simulink model "pv_curves"  (R2024b)
settings: Solver=VariableStepAuto  StartTime=0.0  StopTime=1.0  RelTol=1e-5
libraries: simulink x1, spspowerguiLib x1
settings Model: Creator=jmy  LastModifiedBy=Eng.Abd-Elrhman Saad

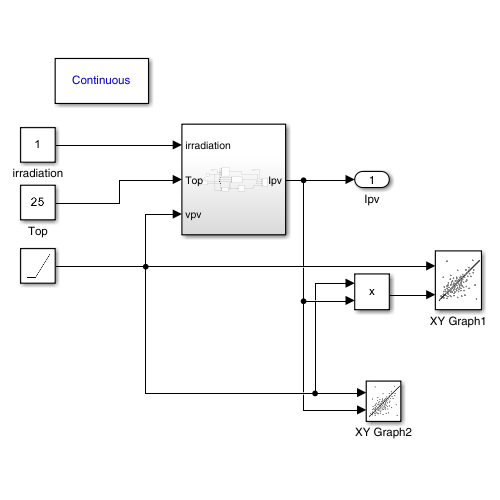
[thumbnail: Simulink's stored preview of the top-level diagram]
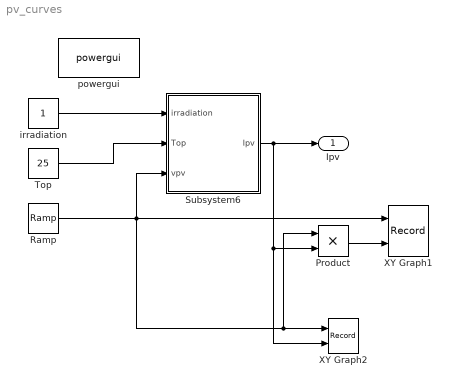
== system pv_curves ==
  Product : Product
  Ramp : simulink/Sources/Ramp  slope=22.9  start=0  InitialOutput=0
  Subsystem6 : Subsystem
  Top : Constant  Value=25
  XY Graph1 : Record  FileSettingsInternal="{\"entries\":[{\"content\":{\"excelSettings\":{\"content\":{},\"type\":\"Streamout.ExcelSettings\"}},\"type\":\"Streamout.FileSettingStorage\",\"uuid\":\"\"}],\"packageUris\":[\"http:\\/\\/schema.mathworks.com\\/mf0\\/streamout_blocks\\/R2020a\"],\"version\":\"1.0\"}"  Layout=[1 1]  SignalsInternal="{\"entries\":[{\"content\":{\"signals\":[{\"content\":{\"blockPath\":[],\"dimensions\":[1],\"domain\":\"\",\"lineColor\":\"#a2142f\",\"plots\":[ 1 ],\"port\":1,\"sid\":[\"\"],\"signalID\":1,\"signalName\":\"Ramp\"},\"type\":\"RecordBlkView.Signal\",\"uuid\":\"\"},{\"content\":{\"blockPath\":[],\"dimensions\":[1],\"domain\":\"\",\"lineColor\":\"#139fff\",\"plots\":[ 1 ],\"port\":2,\"sid\":[\"\"],\"signalID\":2,\"signalName\":\"Product\"},\"type\":\"RecordBlkView.Signal\",\"uuid\":\"\"}]},\"type\":\"RecordBlkView.InputSignals\",\"uuid\":\"\"}],\"packageUris\":[\"http:\\/\\/schema.mathworks.com\\/mf0\\/streamout_blocks\\/R2020a\"],\"version\":\"1.0\"}"  VisualizationBindings="{\"xyplotplugin\":{\"info\":[{\"series\":[{\"bindingParametersList\":[{\"parameter\":\"X-Axis\",\"signalID\":1,\"signalName\":\"Ramp\"},{\"parameter\":\"Y-Axis\",\"signalID\":2,\"signalName\":\"Product\"}],\"seriesID\":0}],\"subplotID\":1}]}}"  CompatibilityTag=XY  st=-1
  XY Graph2 : Record  FileSettingsInternal="{\"entries\":[{\"content\":{\"excelSettings\":{\"content\":{},\"type\":\"Streamout.ExcelSettings\"}},\"type\":\"Streamout.FileSettingStorage\",\"uuid\":\"\"}],\"packageUris\":[\"http:\\/\\/schema.mathworks.com\\/mf0\\/streamout_blocks\\/R2020a\"],\"version\":\"1.0\"}"  Layout=[1 1]  SignalsInternal="{\"entries\":[{\"content\":{\"signals\":[{\"content\":{\"blockPath\":[],\"dimensions\":[1],\"domain\":\"\",\"lineColor\":\"#a2142f\",\"plots\":[ 1 ],\"port\":1,\"sid\":[\"\"],\"signalID\":1,\"signalName\":\"Ramp\"},\"type\":\"RecordBlkView.Signal\",\"uuid\":\"\"},{\"content\":{\"blockPath\":[],\"dimensions\":[1],\"domain\":\"\",\"lineColor\":\"#139fff\",\"plots\":[ 1 ],\"port\":2,\"sid\":[\"\"],\"signalID\":2,\"signalName\":\"Subsystem6\"},\"type\":\"RecordBlkView.Signal\",\"uuid\":\"\"}]},\"type\":\"RecordBlkView.InputSignals\",\"uuid\":\"\"}],\"packageUris\":[\"http:\\/\\/schema.mathworks.com\\/mf0\\/streamout_blocks\\/R2020a\"],\"version\":\"1.0\"}"  VisualizationBindings="{\"xyplotplugin\":{\"info\":[{\"series\":[{\"bindingParametersList\":[{\"parameter\":\"X-Axis\",\"signalID\":1,\"signalName\":\"Ramp\"},{\"parameter\":\"Y-Axis\",\"signalID\":2,\"signalName\":\"Subsystem6\"}],\"seriesID\":0}],\"subplotID\":1}]}}"  CompatibilityTag=XY  st=-1
  irradiation : Constant
  powergui : spspowerguiLib/powergui  Priority=1  SimulationMode=Continuous  SampleTime=50e-6  frequency=60  Iterations=50  frequencyindice=60  Pbase=100e6  ErrMax=1e-4  UnitsV=kV  UnitsW=MW  buscounter=0  FunctionMessages=off  echomessages=off  EnableUseOfTLC=off  CurrentSourceSwitches=off  DisableSnubberDevices=off  DisableRonSwitches=off  DisableVfSwitches=off  DisplayEquations=off  AutomaticDiscreteSolvers=off  SolverType=Tustin/Backward Euler (TBE)  Interpol=off  ExternalGateDelay=off  methode=off  Ts=100  x0status=blocks  SPID=on  SwTol=0  HookPort=off  NonlinearTolerance=1e-4  nMaxIteration=100  ContinueOnMaxIteration=off  RestoreLinks=warning  ResistiveCurrentMeasurement=off  Frange=[0:2:500]  Ylog=off  Xlog=on  ShowGrid=off  save=off  variable=ZData  structure=0  ZoomFFT=off  StartTime=0.0  cycles=1  DisplayStyle=1  fundamental=60  FreqAxis=off  MaxFrequency=1000  frequencyindicesteady=1  RmsSteady=1  display=off
  Ipv : Outport
  wires:
  irradiation/1 -> Subsystem6/1(irradiation)
  Top/1 -> Subsystem6/2(Top)
  Ramp/1 -> XY Graph2/1, Product/1, Subsystem6/3(vpv), XY Graph1/1
  Subsystem6/1(Ipv) -> Product/2, XY Graph2/2, Ipv/1
  Product/1 -> XY Graph1/2

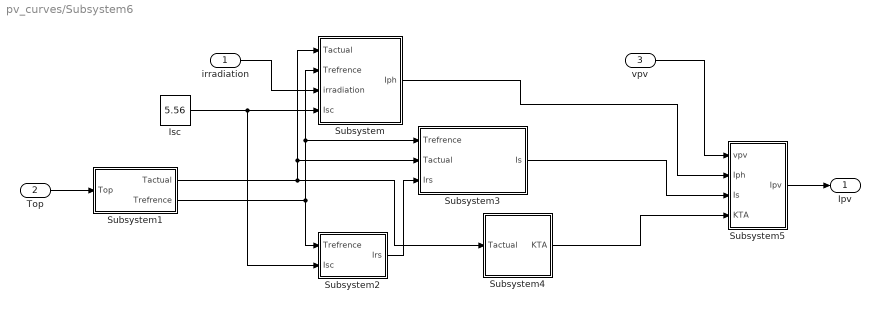
== system pv_curves/Subsystem6 ==
  irradiation : Inport
  Top : Inport  Port=2
  vpv : Inport  Port=3
  Isc : Constant  Value=5.56
  Subsystem : Subsystem
  Subsystem1 : Subsystem
  Subsystem2 : Subsystem
  Subsystem3 : Subsystem
  Subsystem4 : Subsystem
  Subsystem5 : Subsystem
  Ipv : Outport
  wires:
  Isc/1 -> Subsystem2/2(Isc), Subsystem/4(Isc)
  Subsystem1/2(Trefrence) -> Subsystem/2(Trefrence), Subsystem3/1(Trefrence), Subsystem2/1(Trefrence)
  Top/1 -> Subsystem1/1(Top)
  irradiation/1 -> Subsystem/3(irradiation)
  Subsystem4/1(KTA) -> Subsystem5/4(KTA)
  Subsystem1/1(Tactual) -> Subsystem4/1(Tactual), Subsystem3/2(Tactual), Subsystem/1(Tactual)
  vpv/1 -> Subsystem5/1(vpv)
  Subsystem3/1(Is) -> Subsystem5/3(Is)
  Subsystem2/1(Irs) -> Subsystem3/3(Irs)
  Subsystem/1(Iph) -> Subsystem5/2(Iph)
  Subsystem5/1(Ipv) -> Ipv/1

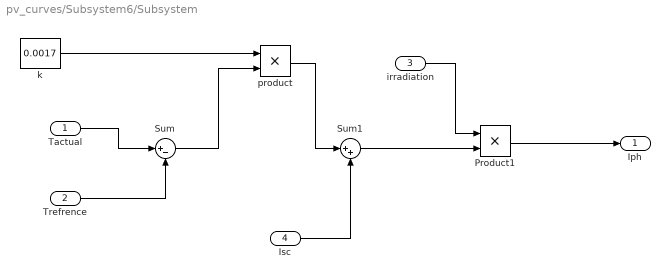
== system pv_curves/Subsystem6/Subsystem ==
  Tactual : Inport
  Trefrence : Inport  Port=2
  irradiation : Inport  Port=3
  Isc : Inport  Port=4
  Product1 : Product
  Sum : Sum  Inputs=|+-
  Sum1 : Sum  Inputs=|++
  k : Constant  Value=0.0017
  product : Product
  Iph : Outport
  wires:
  irradiation/1 -> Product1/1
  Sum/1 -> product/2
  Isc/1 -> Sum1/2
  Trefrence/1 -> Sum/2
  product/1 -> Sum1/1
  Sum1/1 -> Product1/2
  k/1 -> product/1
  Product1/1 -> Iph/1
  Tactual/1 -> Sum/1

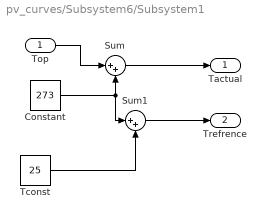
== system pv_curves/Subsystem6/Subsystem1 ==
  Top : Inport
  Constant : Constant  Value=273
  Sum : Sum  Inputs=|++
  Sum1 : Sum  Inputs=|++
  Tconst : Constant  Value=25
  Tactual : Outport
  Trefrence : Outport  Port=2
  wires:
  Constant/1 -> Sum1/1, Sum/2
  Sum1/1 -> Trefrence/1
  Top/1 -> Sum/1
  Tconst/1 -> Sum1/2
  Sum/1 -> Tactual/1

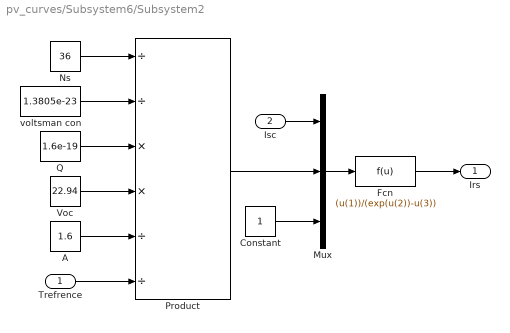
== system pv_curves/Subsystem6/Subsystem2 ==
  Trefrence : Inport
  Isc : Inport  Port=2
  A : Constant  Value=1.6
  Constant : Constant
  Fcn : Fcn  Expr=(u(1))/(exp(u(2))-u(3))
  Mux : Mux  Inputs=3
  Ns : Constant  Value=36
  Product : Product  Inputs=//**//
  Q : Constant  Value=1.6e-19
  Voc : Constant  Value=22.94
  voltsman con : Constant  Value=1.3805e-23
  Irs : Outport
  wires:
  Voc/1 -> Product/4
  Ns/1 -> Product/1
  A/1 -> Product/5
  Mux/1 -> Fcn/1
  voltsman con/1 -> Product/2
  Constant/1 -> Mux/3
  Trefrence/1 -> Product/6
  Q/1 -> Product/3
  Isc/1 -> Mux/1
  Product/1 -> Mux/2
  Fcn/1 -> Irs/1

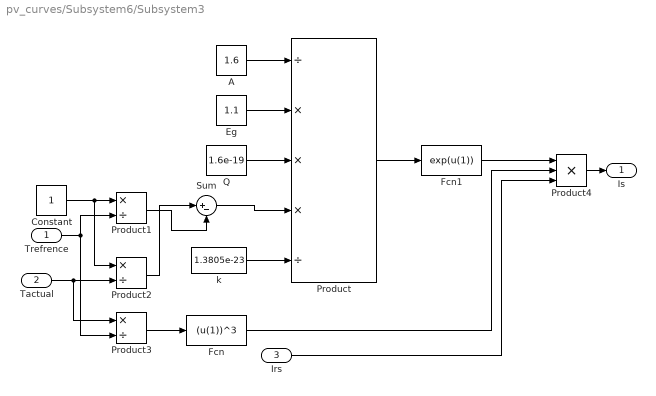
== system pv_curves/Subsystem6/Subsystem3 ==
  Trefrence : Inport
  Tactual : Inport  Port=2
  Irs : Inport  Port=3
  A : Constant  Value=1.6
  Constant : Constant
  Eg : Constant  Value=1.1
  Fcn : Fcn  Expr=(u(1))^3
  Fcn1 : Fcn  Expr=exp(u(1))
  Product : Product  Inputs=/***/
  Product1 : Product  Inputs=*/
  Product2 : Product  Inputs=*/
  Product3 : Product  Inputs=*/
  Product4 : Product  Inputs=3
  Q : Constant  Value=1.6e-19
  Sum : Sum  Inputs=|+-
  k : Constant  Value=1.3805e-23
  Is : Outport
  wires:
  A/1 -> Product/1
  Eg/1 -> Product/2
  Trefrence/1 -> Product3/2, Product1/2
  k/1 -> Product/5
  Constant/1 -> Product2/1, Product1/1
  Irs/1 -> Product4/3
  Tactual/1 -> Product3/1, Product2/2
  Product3/1 -> Fcn/1
  Sum/1 -> Product/4
  Q/1 -> Product/3
  Fcn/1 -> Product4/2
  Product4/1 -> Is/1
  Product1/1 -> Sum/2
  Product2/1 -> Sum/1
  Product/1 -> Fcn1/1
  Fcn1/1 -> Product4/1

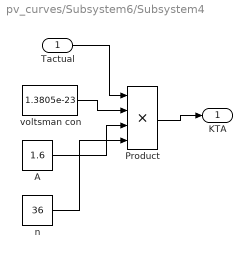
== system pv_curves/Subsystem6/Subsystem4 ==
  Tactual : Inport
  A : Constant  Value=1.6
  Product : Product  Inputs=4
  n : Constant  Value=36
  voltsman con : Constant  Value=1.3805e-23
  KTA : Outport
  wires:
  Tactual/1 -> Product/1
  voltsman con/1 -> Product/2
  A/1 -> Product/3
  Product/1 -> KTA/1
  n/1 -> Product/4

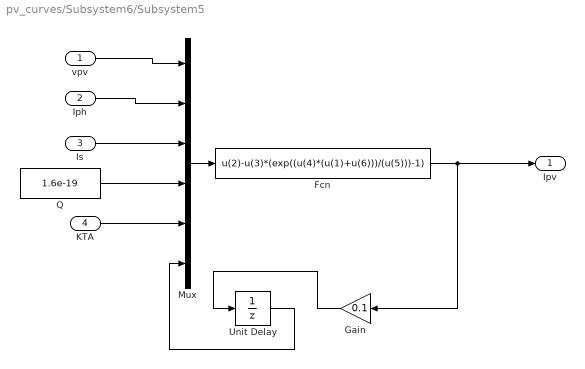
== system pv_curves/Subsystem6/Subsystem5 ==
  vpv : Inport
  Iph : Inport  Port=2
  Is : Inport  Port=3
  KTA : Inport  Port=4
  Fcn : Fcn  Expr=u(2)-u(3)*(exp((u(4)*(u(1)+u(6)))/(u(5)))-1)
  Gain : Gain  Gain=0.1
  Mux : Mux  Inputs=6
  Q : Constant  Value=1.6e-19
  Unit Delay : UnitDelay  SampleTime=-1  HasFrameUpgradeWarning=on
  Ipv : Outport
  wires:
  Iph/1 -> Mux/2
  Mux/1 -> Fcn/1
  Fcn/1 -> Gain/1, Ipv/1
  vpv/1 -> Mux/1
  KTA/1 -> Mux/5
  Is/1 -> Mux/3
  Q/1 -> Mux/4
  Unit Delay/1 -> Mux/6
  Gain/1 -> Unit Delay/1
